simulink model "flightSim_Simulink"  (R2025b)
settings: Solver=VariableStepAuto  StartTime=0.0  StopTime=200  FixedStep=1/120  RelTol=1e-5
model workspace (MATLAB code in the model file):
  | initialize6DOFSkyHogg;
values from neighbouring files (symbols this model uses):
  aircraft = aircraft.update()    [flightSim_createAircraft.m]    (also in in_class_createAircraft.m)
  control = @(alpha, q) K_alpha*(alpha_desired - alpha) + K_q*(q_desired - q)    [sp_cntrl_ex.m]
  q = rate(2,itr)    [in_class_coding.m]    (also in in_class_sp_control.m = x(2,i); rigidBodyModel.m = rate(2); sp_cntrl_ex.m = xx(2,i))
  r = rate(3,itr)    [in_class_coding.m]    (also in rigidBodyModel.m = rate(3))
  state = fixedWingState(aircraft, Environment)    [flightSim_createAircraft.m]    (also in in_class_createAircraft.m)
undefined symbols (not defined in the file or in its folder): F, Light, MIL
libraries: aerolibasang x5, aerolibobsolete x1, aerolibadyn x1, aerolibatmos2 x1, aerolibwind2 x1, sharedtransform x1
settings Model: Creator=User  LastModifiedBy=tkhamvil
settings SolverCC: AlgebraicLoopSolver=TrustRegion  AutoInsertRateTranBlk=on  InsertRTBMode=Never (minimum delay)  MinimalZcImpactIntegration=on  MaxZcPerStep=1.0
settings DataIOCC: ExternalInput=inputs0  InitialState=states  SaveFormat=Array  SaveOutput=off
settings OptimizationCC: EnhancedBackFolding=on  StrengthReduction=on  InitFltsAndDblsToZero=on  DifferentSizesBufferReuse=on
settings DebuggingCC: WriteAfterWriteMsg=DisableAll  AlgebraicLoopMsg=none  FcnCallInpInsideContextMsg=warning  UniqueDataStoreMsg=error  RootOutportRequireBusObject=none  StateNameClashWarn=warning  StrictBusMsg=ErrorOnBusTreatedAsVector  SFUnexpectedBacktrackingDiag=warning  SFNoUnconditionalDefaultTransitionDiag=warning  SFExecutionAtInitializationDiag=none  ArithmeticOperatorsInVariantConditions=warning
settings ModelReferenceCC: EnableRefExpFcnMdlSchedulingChecks=on  PropagateSignalLabelsOutOfModel=off
settings SFSimCC: SimUseLocalCustomCode=off
settings RTWCC: RTWUseLocalCustomCode=off  GPUComputeCapability=3.5  DLArmComputeVersion=19.05
settings CodeAppCC: StateflowObjectComments=on

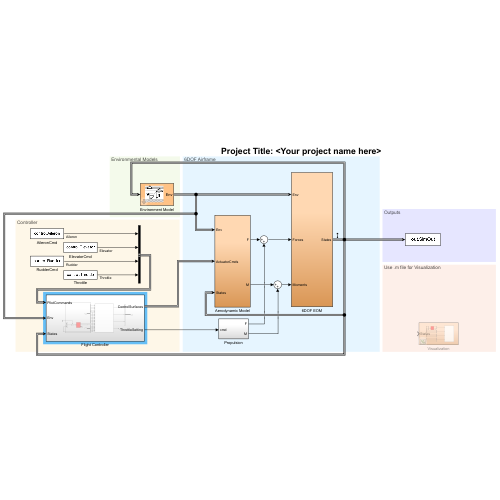
[thumbnail: Simulink's stored preview of the top-level diagram]
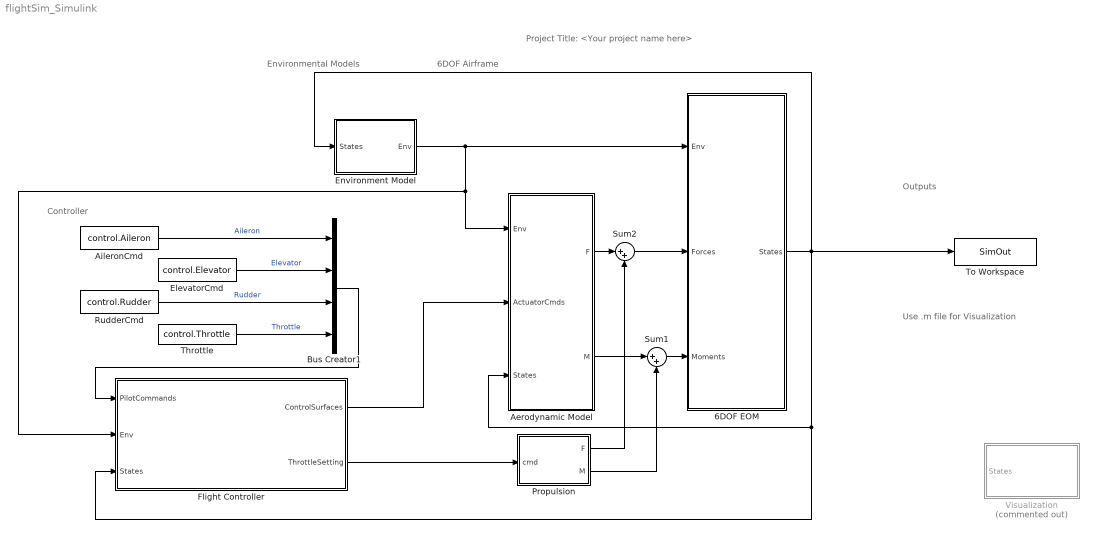
== system flightSim_Simulink ==
  note: Project Title: <Your project name here>
  note: 6DOF Airframe
  note: Environmental Models
  note: Controller
  note: Use .m file for Visualization
  note: Outputs
  6DOF EOM : Subsystem  VariantControl=eom3DOF
  Aerodynamic Model : Subsystem  VariantControl=aeroCONST
  AileronCmd : Constant  Value=control.Aileron
  Bus Creator1 : BusCreator  Inputs=4
  ElevatorCmd : Constant  Value=control.Elevator
  Environment Model : Subsystem  mask(Environment Model){spec=MIL-F-8785C, model=Continuous Dryden (+q -r), W20=5, Wdeg=0, TurbProb=10^-2 - Light, L_high=533.4, Wingspan=4, ts=0.1, Seed=[23341 23342 23343 23344], T_on=off, refAlt=state.GroundHeight}
      mask prompts: spec "aeroblks:aeroblkwind:blockWindTurbulenceModelParamSpecification"; model "aeroblks:aeroblkwind:blockWindTurbulenceModelParamModeltype"; W20 "Wind speed at 6 m defines the low-altitude intensity (m/s):"; Wdeg "Wind direction at 6 m (degrees clockwise from north):"; TurbProb "aeroblks:aeroblkwind:blockWindTurbulenceModelParamProbabilityofexceedanceofhighaltitudeintensity"; L_high "Scale length at medium/high altitudes (m):"; Wingspan "Wingspan (m):"; ts "Band limited noise sample time (sec):"; Seed "aeroblks:aeroblkwind:blockWindTurbulenceModelParamNoiseseedsugvgwgpg"; T_on "aeroblks:aeroblkwind:blockWindTurbulenceModelParamTurbulenceon"; refAlt "Reference height from Earth's surface to Flat Earth frame [m]:"
      mask help: This block contains an athmospheric model, a wind turbulence model, and a gravity model.
      mask Help: helpview(fullfile(docroot,'toolbox','aeroblks','aeroblks.map'), 'environment1');
      mask TypeOptions spec:
      | Dryden Wind Turbulence Model
      | (Continuous (+q +r))/spec
      mask TypeOptions model:
      | Dryden Wind Turbulence Model
      | (Continuous (+q +r))/model
      mask TypeOptions W20:
      | Dryden Wind Turbulence Model
      | (Continuous (+q +r))/W20
      mask TypeOptions Wdeg:
      | Dryden Wind Turbulence Model
      | (Continuous (+q +r))/Wdeg
      mask TypeOptions TurbProb:
      | Dryden Wind Turbulence Model
      | (Continuous (+q +r))/TurbProb
      mask TypeOptions L_high:
      | Dryden Wind Turbulence Model
      | (Continuous (+q +r))/L_high
      mask TypeOptions Wingspan:
      | Dryden Wind Turbulence Model
      | (Continuous (+q +r))/Wingspan
      mask TypeOptions ts:
      | Dryden Wind Turbulence Model
      | (Continuous (+q +r))/ts
      mask TypeOptions Seed:
      | Dryden Wind Turbulence Model
      | (Continuous (+q +r))/Seed
      mask TypeOptions T_on:
      | Dryden Wind Turbulence Model
      | (Continuous (+q +r))/T_on
      mask DialogControl Container4 Prompt: Atmospheric Model
      mask DialogControl Container17 Prompt: 1976 COESA-extended U.S. Standard Atmospheric Model
      mask DialogControl Control6 Prompt: There are no modifiable parameters for COESA.
      mask DialogControl Container6 Prompt: Wind Model
      mask DialogControl Container16 Prompt: Dryden Wind Turbulence Model
      mask DialogControl spec Prompt: Specification:
      mask DialogControl model Prompt: Model type:
      mask DialogControl TurbProb Prompt: Probability of exceedance of high-altitude intensity:
      mask DialogControl Seed Prompt: Noise seeds [ug vg wg pg]:
      mask DialogControl T_on Prompt: Turbulence on
      mask DialogControl Container8 Prompt: Gravity Model
      mask DialogControl Container18 Prompt: World Geodetic System (WGS 84) Gravity Taylor Series Model
      mask Display:
      | image('aeroenvironment.bmp',[.15,.15,.55,.75])
      | port_label('output',1,'Env')
  Flight Controller : Subsystem
  Propulsion : Subsystem
      settings: RTWSystemCode=Inline
  RudderCmd : Constant  Value=control.Rudder
  Sum1 : Sum  Inputs=|++  InputSameDT=on  SaturateOnIntegerOverflow=on  OutDataTypeStr=Inherit: Same as first input
  Sum2 : Sum  Inputs=|++  InputSameDT=on  SaturateOnIntegerOverflow=on  OutDataTypeStr=Inherit: Same as first input
  Throttle : Constant  Value=control.Throttle
  To Workspace : ToWorkspace  VariableName=SimOut  SaveFormat=Timeseries  SampleTime=-1
  Visualization : Subsystem  Commented=on
  wires:
  Sum2/1 -> 6DOF EOM/2(Forces)
  Propulsion/2(M) -> Sum1/2
  Propulsion/1(F) -> Sum2/2
  Sum1/1 -> 6DOF EOM/3(Moments)
  Aerodynamic Model/1(F) -> Sum2/1
  Aerodynamic Model/2(M) -> Sum1/1
  Environment Model/1(Env) -> Aerodynamic Model/1(Env), Flight Controller/2(Env), 6DOF EOM/1(Env)
  6DOF EOM/1(States) -> Flight Controller/3(States), Aerodynamic Model/3(States), To Workspace/1, Environment Model/1(States)
  Flight Controller/1(ControlSurfaces) -> Aerodynamic Model/2(ActuatorCmds)
  Flight Controller/2(ThrottleSetting) -> Propulsion/1(cmd)
  AileronCmd/1 -> Bus Creator1/1  "Aileron"
  ElevatorCmd/1 -> Bus Creator1/2  "Elevator"
  RudderCmd/1 -> Bus Creator1/3  "Rudder"
  Throttle/1 -> Bus Creator1/4  "Throttle"
  Bus Creator1/1 -> Flight Controller/1(PilotCommands)

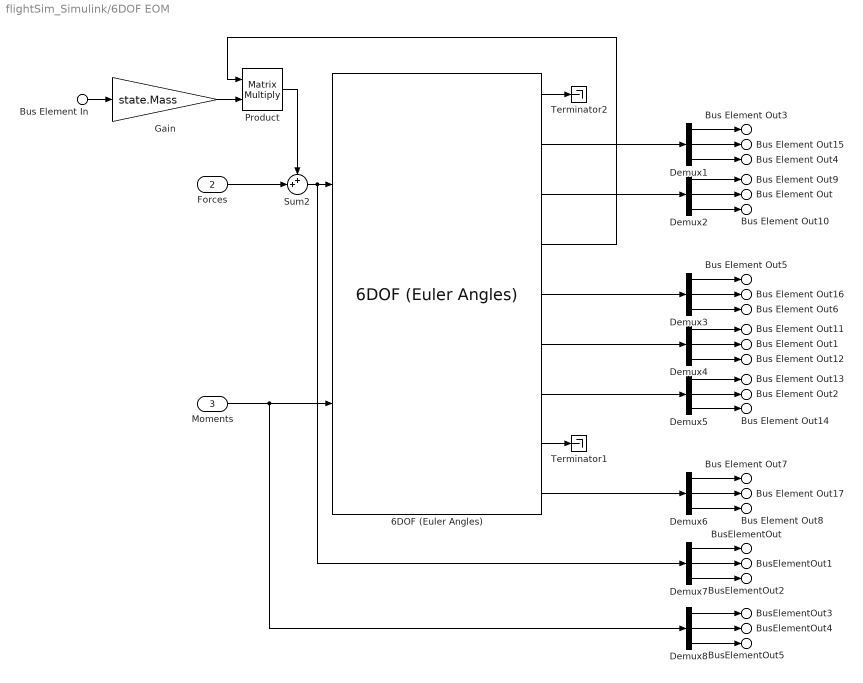
== system flightSim_Simulink/6DOF EOM ==
  Bus Element In : Inport  PortName=Env  Element=g
  Forces : Inport  Port=2
  Moments : Inport  Port=3
  6DOF (Euler Angles) : aerolibobsolete/6DOF (Euler Angles)  units=Metric (MKS)  mtype=Fixed  rep=Euler Angles  xme_0=[state.XN, state.XE, state.XD]  Vm_0=[state.U, state.V, state.W]  eul_0=[state.Phi, state.Theta, state.Psi]  pm_0=[state.P, state.Q, state.R]  mass_0=state.Mass  mass_e=0.5  mass_f=2.0  inertia=state.Inertia.Variables  inertia_e=eye(3)  inertia_f=2*eye(3)  k_quat=1.0  vre_flag=on  abi_flag=on  aMode=0  xme_statename={'Xe', 'Ye', 'Ze'}  Vm_statename={'U', 'V', 'W'}  eul_statename={'phi', 'theta', 'psi'}  quat_statename={'qr', 'qi', 'qj','qk'}  pm_statename={'p', 'q', 'r'}  mass_statename=''
  Demux{1..8} (8 alike) : Demux  Outputs=3
  Gain : Gain  Gain=state.Mass
  Product : Product  Multiplication=Matrix(*)
  Sum2 : Sum  Inputs=++|  InputSameDT=on  SaturateOnIntegerOverflow=on  OutDataTypeStr=Inherit: Same as first input
  Terminator1 : Terminator
  Terminator2 : Terminator
  Bus Element Out3 : Outport  VectorParamsAs1DForOutWhenUnconnected=off  PortName=States  Element=Xe
  Bus Element Out4 : Outport  VectorParamsAs1DForOutWhenUnconnected=off  PortName=States  Element=Ze
  Bus Element Out : Outport  VectorParamsAs1DForOutWhenUnconnected=off  PortName=States  Element=theta
  Bus Element Out5 : Outport  VectorParamsAs1DForOutWhenUnconnected=off  PortName=States  Element=u
  Bus Element Out6 : Outport  VectorParamsAs1DForOutWhenUnconnected=off  PortName=States  Element=w
  Bus Element Out1 : Outport  VectorParamsAs1DForOutWhenUnconnected=off  PortName=States  Element=q
  Bus Element Out2 : Outport  VectorParamsAs1DForOutWhenUnconnected=off  PortName=States  Element=q_dot
  Bus Element Out7 : Outport  VectorParamsAs1DForOutWhenUnconnected=off  PortName=States  Element=Axe
  Bus Element Out8 : Outport  VectorParamsAs1DForOutWhenUnconnected=off  PortName=States  Element=Aze
  Bus Element Out15 : Outport  VectorParamsAs1DForOutWhenUnconnected=off  PortName=States  Element=Ye
  Bus Element Out9 : Outport  VectorParamsAs1DForOutWhenUnconnected=off  PortName=States  Element=phi
  Bus Element Out10 : Outport  VectorParamsAs1DForOutWhenUnconnected=off  PortName=States  Element=psi
  Bus Element Out16 : Outport  VectorParamsAs1DForOutWhenUnconnected=off  PortName=States  Element=v
  Bus Element Out11 : Outport  VectorParamsAs1DForOutWhenUnconnected=off  PortName=States  Element=p
  Bus Element Out12 : Outport  VectorParamsAs1DForOutWhenUnconnected=off  PortName=States  Element=r
  Bus Element Out13 : Outport  VectorParamsAs1DForOutWhenUnconnected=off  PortName=States  Element=p_dot
  Bus Element Out14 : Outport  VectorParamsAs1DForOutWhenUnconnected=off  PortName=States  Element=r_dot
  Bus Element Out17 : Outport  VectorParamsAs1DForOutWhenUnconnected=off  PortName=States  Element=Aye
  BusElementOut : Outport  PortName=States  Element=X
  BusElementOut1 : Outport  PortName=States  Element=Y
  BusElementOut2 : Outport  PortName=States  Element=Z
  BusElementOut3 : Outport  PortName=States  Element=L
  BusElementOut4 : Outport  PortName=States  Element=M
  BusElementOut5 : Outport  PortName=States  Element=N
  wires:
  6DOF (Euler Angles)/2 -> Demux1/1
  6DOF (Euler Angles)/4 -> Product/1
  6DOF (Euler Angles)/1 -> Terminator2/1
  Bus Element In/1 -> Gain/1
  Demux6/2 -> Bus Element Out17/1
  Demux6/3 -> Bus Element Out8/1
  Demux6/1 -> Bus Element Out7/1
  6DOF (Euler Angles)/9 -> Demux6/1
  6DOF (Euler Angles)/7 -> Demux5/1
  Demux5/3 -> Bus Element Out14/1
  Demux5/2 -> Bus Element Out2/1
  Demux5/1 -> Bus Element Out13/1
  6DOF (Euler Angles)/6 -> Demux4/1
  Demux4/3 -> Bus Element Out12/1
  Demux4/2 -> Bus Element Out1/1
  Demux4/1 -> Bus Element Out11/1
  Demux3/3 -> Bus Element Out6/1
  Demux3/2 -> Bus Element Out16/1
  Demux3/1 -> Bus Element Out5/1
  6DOF (Euler Angles)/5 -> Demux3/1
  Demux2/3 -> Bus Element Out10/1
  Demux2/2 -> Bus Element Out/1
  Demux2/1 -> Bus Element Out9/1
  Demux1/1 -> Bus Element Out3/1
  Demux1/3 -> Bus Element Out4/1
  Demux1/2 -> Bus Element Out15/1
  Gain/1 -> Product/2
  6DOF (Euler Angles)/3 -> Demux2/1
  Forces/1 -> Sum2/2
  Product/1 -> Sum2/1
  6DOF (Euler Angles)/8 -> Terminator1/1
  Sum2/1 -> Demux7/1, 6DOF (Euler Angles)/1
  Moments/1 -> Demux8/1, 6DOF (Euler Angles)/2
  Demux7/1 -> BusElementOut/1
  Demux7/2 -> BusElementOut1/1
  Demux7/3 -> BusElementOut2/1
  Demux8/1 -> BusElementOut3/1
  Demux8/2 -> BusElementOut4/1
  Demux8/3 -> BusElementOut5/1

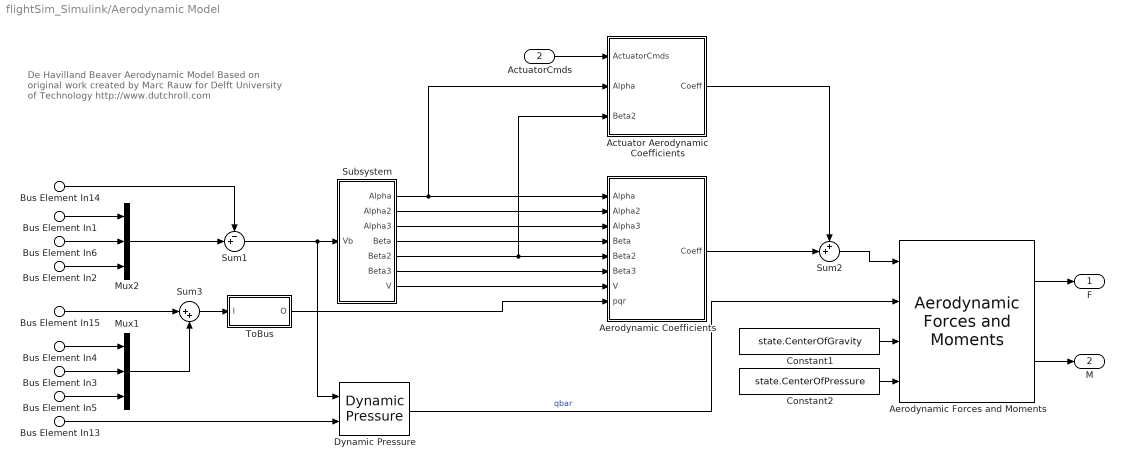
== system flightSim_Simulink/Aerodynamic Model ==
  note: De Havilland Beaver Aerodynamic Model
      | Based on original work created by
      | Marc Rauw for Delft University of Technology
      | http://www.dutchroll.com
  Bus Element In13 : Inport  PortName=Env  Element=AirDensity
  Bus Element In14 : Inport  PortName=Env  Element=WindVelocity
  Bus Element In15 : Inport  PortName=Env  Element=WindAngularRates
  ActuatorCmds : Inport  Port=2
  Bus Element In1 : Inport  Port=3  PortName=States  Element=u
  Bus Element In2 : Inport  Port=3  PortName=States  Element=w
  Bus Element In3 : Inport  Port=3  PortName=States  Element=q
  Bus Element In6 : Inport  Port=3  PortName=States  Element=v
  Bus Element In4 : Inport  Port=3  PortName=States  Element=p
  Bus Element In5 : Inport  Port=3  PortName=States  Element=r
  Actuator Aerodynamic Coefficients : Subsystem
  Aerodynamic Coefficients : Subsystem
  Aerodynamic Forces and Moments : aerolibadyn/Aerodynamic Forces and Moments   inputAxes=Body  outputForceAxes=Body  outputMomentAxes=Body  S=aircraft.ReferenceArea  b=aircraft.ReferenceSpan  cbar=aircraft.ReferenceLength
  Constant1 : Constant  Value=state.CenterOfGravity
  Constant2 : Constant  Value=state.CenterOfPressure
  Dynamic Pressure : aerolibasang/Dynamic Pressure
  Mux1 : Mux  Inputs=3
  Mux2 : Mux  Inputs=3
  Subsystem : Subsystem
  Sum1 : Sum  Inputs=-+|  InputSameDT=on  SaturateOnIntegerOverflow=on  OutDataTypeStr=Inherit: Same as first input
  Sum2 : Sum  Inputs=++|
  Sum3 : Sum  Inputs=|++  InputSameDT=on  SaturateOnIntegerOverflow=on  OutDataTypeStr=Inherit: Same as first input
  ToBus : Subsystem
  F : Outport  Unit=N  VectorParamsAs1DForOutWhenUnconnected=off
  M : Outport  Port=2  Unit=N*m  VectorParamsAs1DForOutWhenUnconnected=off
  wires:
  ActuatorCmds/1 -> Actuator Aerodynamic Coefficients/1(ActuatorCmds)
  Bus Element In14/1 -> Sum1/1
  Mux2/1 -> Sum1/2
  Mux1/1 -> Sum3/2
  Bus Element In15/1 -> Sum3/1
  Bus Element In5/1 -> Mux1/3
  Bus Element In3/1 -> Mux1/2
  Bus Element In4/1 -> Mux1/1
  Actuator Aerodynamic Coefficients/1(Coeff) -> Sum2/1
  Aerodynamic Coefficients/1(Coeff) -> Sum2/2
  ToBus/1(O) -> Aerodynamic Coefficients/8(pqr)
  Sum1/1 -> Dynamic Pressure/1, Subsystem/1(Vb)
  Dynamic Pressure/1 -> Aerodynamic Forces and Moments/2  "qbar"
  Sum3/1 -> ToBus/1(I)
  Bus Element In13/1 -> Dynamic Pressure/2
  Subsystem/7(V) -> Aerodynamic Coefficients/7(V)
  Subsystem/4(Beta) -> Aerodynamic Coefficients/4(Beta)
  Aerodynamic Forces and Moments/2 -> M/1
  Aerodynamic Forces and Moments/1 -> F/1
  Constant2/1 -> Aerodynamic Forces and Moments/4
  Constant1/1 -> Aerodynamic Forces and Moments/3
  Sum2/1 -> Aerodynamic Forces and Moments/1
  Bus Element In1/1 -> Mux2/1
  Bus Element In6/1 -> Mux2/2
  Bus Element In2/1 -> Mux2/3
  Subsystem/1(Alpha) -> Aerodynamic Coefficients/1(Alpha), Actuator Aerodynamic Coefficients/2(Alpha)
  Subsystem/5(Beta2) -> Aerodynamic Coefficients/5(Beta2), Actuator Aerodynamic Coefficients/3(Beta2)
  Subsystem/2(Alpha2) -> Aerodynamic Coefficients/2(Alpha2)
  Subsystem/3(Alpha3) -> Aerodynamic Coefficients/3(Alpha3)
  Subsystem/6(Beta3) -> Aerodynamic Coefficients/6(Beta3)

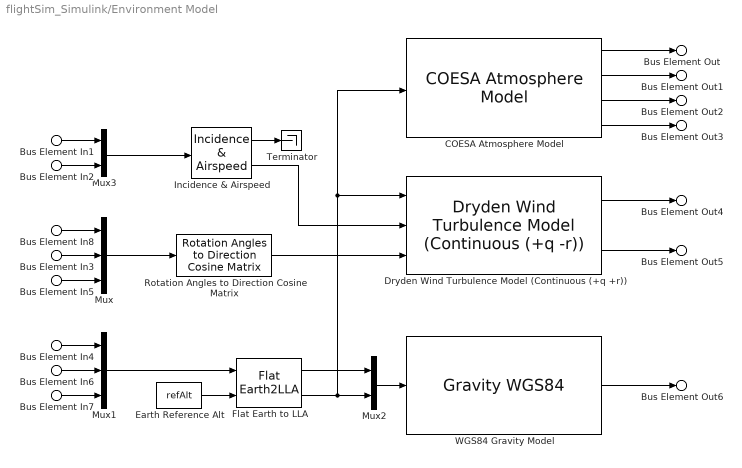
== system flightSim_Simulink/Environment Model ==
  Bus Element In1 : Inport  PortName=States  Element=u
  Bus Element In2 : Inport  PortName=States  Element=w
  Bus Element In3 : Inport  PortName=States  Element=theta
  Bus Element In4 : Inport  PortName=States  Element=Xe
  Bus Element In7 : Inport  PortName=States  Element=Ze
  Bus Element In8 : Inport  PortName=States  Element=phi
  Bus Element In5 : Inport  PortName=States  Element=psi
  Bus Element In6 : Inport  PortName=States  Element=Ye
  COESA Atmosphere Model : aerolibatmos2/COESA Atmosphere Model  units=Metric (MKS)  spec=1976 COESA-extended U.S. Standard Atmosphere  model=Profile  profile_var=High temperature  profile_percent=1%  profile_alt=5 km (16404 ft)  envelope_var=High temperature  envelope_percent=1%  action=Warning
  Dryden Wind Turbulence Model (Continuous (+q +r)) : aerolibwind2/Dryden Wind Turbulence Model  (Continuous (+q -r))  units=Metric (MKS)  spec=MIL-F-8785C  model=Continuous Dryden (+q -r)  W20=W20  Wdeg=Wdeg  TurbProb=10^-2 - Light  L_high=L_high  Wingspan=Wingspan  ts=ts  Seed=Seed  T_on=off
  Earth Reference Alt : Constant  Value=refAlt
  Flat Earth to LLA : FlatEarth2LLA  R=6378137  LL0=[0 0]
  Incidence & Airspeed : aerolibasang/Incidence  & Airspeed
  Mux : Mux  Inputs=3
  Mux1 : Mux  Inputs=3
  Mux2 : Mux  Inputs=2
  Mux3 : Mux  Inputs=2
  Rotation Angles to Direction Cosine Matrix : sharedtransform/Rotation Angles to Direction Cosine Matrix  rotationOrder=ZYX  aMode=aMode
  Terminator : Terminator
  "WGS84 Gravity Model  " : GravityWGS84
  Bus Element Out : Outport  VectorParamsAs1DForOutWhenUnconnected=off  PortName=Env  Element=To
  Bus Element Out1 : Outport  VectorParamsAs1DForOutWhenUnconnected=off  PortName=Env  Element=a
  Bus Element Out2 : Outport  VectorParamsAs1DForOutWhenUnconnected=off  PortName=Env  Element=Po
  Bus Element Out3 : Outport  VectorParamsAs1DForOutWhenUnconnected=off  PortName=Env  Element=AirDensity
  Bus Element Out4 : Outport  VectorParamsAs1DForOutWhenUnconnected=off  PortName=Env  Element=WindVelocity
  Bus Element Out5 : Outport  VectorParamsAs1DForOutWhenUnconnected=off  PortName=Env  Element=WindAngularRates
  Bus Element Out6 : Outport  VectorParamsAs1DForOutWhenUnconnected=off  PortName=Env  Element=g
  wires:
  Dryden Wind Turbulence Model (Continuous (+q +r))/1 -> Bus Element Out4/1
  Dryden Wind Turbulence Model (Continuous (+q +r))/2 -> Bus Element Out5/1
  Mux2/1 -> "WGS84 Gravity Model  "/1
  Bus Element In4/1 -> Mux1/1
  Bus Element In7/1 -> Mux1/3
  Bus Element In6/1 -> Mux1/2
  Bus Element In5/1 -> Mux/3
  Bus Element In8/1 -> Mux/1
  Bus Element In2/1 -> Mux3/2
  Bus Element In1/1 -> Mux3/1
  "WGS84 Gravity Model  "/1 -> Bus Element Out6/1
  COESA Atmosphere Model/2 -> Bus Element Out1/1
  COESA Atmosphere Model/1 -> Bus Element Out/1
  COESA Atmosphere Model/4 -> Bus Element Out3/1
  COESA Atmosphere Model/3 -> Bus Element Out2/1
  Flat Earth to LLA/1 -> Mux2/1
  Earth Reference Alt/1 -> Flat Earth to LLA/2
  Incidence & Airspeed/2 -> Dryden Wind Turbulence Model (Continuous (+q +r))/2
  Flat Earth to LLA/2 -> Mux2/2, COESA Atmosphere Model/1, Dryden Wind Turbulence Model (Continuous (+q +r))/1
  Mux3/1 -> Incidence & Airspeed/1
  Incidence & Airspeed/1 -> Terminator/1
  Mux/1 -> Rotation Angles to Direction Cosine Matrix/1
  Bus Element In3/1 -> Mux/2
  Rotation Angles to Direction Cosine Matrix/1 -> Dryden Wind Turbulence Model (Continuous (+q +r))/3
  Mux1/1 -> Flat Earth to LLA/1

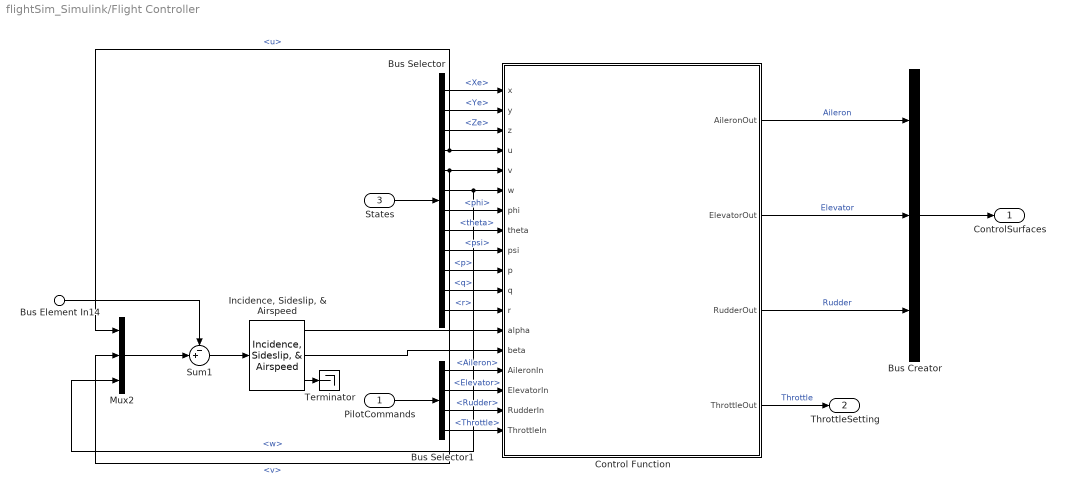
== system flightSim_Simulink/Flight Controller ==
  PilotCommands : Inport
  Bus Element In14 : Inport  Port=2  PortName=Env  Element=WindVelocity
  States : Inport  Port=3
  Bus Creator : BusCreator  Inputs=3
  Bus Selector : BusSelector  OutputSignals=Xe,Ye,Ze,u,v,w,phi,theta,psi,p,q,r
  Bus Selector1 : BusSelector  OutputSignals=Aileron,Elevator,Rudder,Throttle
  Control Function : MATLAB Function  TreatAsAtomicUnit=on
  "Incidence, Sideslip, & Airspeed" : aerolibasang/Incidence, Sideslip, & Airspeed
  Mux2 : Mux  Inputs=3
  Sum1 : Sum  Inputs=-+|  InputSameDT=on  SaturateOnIntegerOverflow=on  OutDataTypeStr=Inherit: Same as first input
  Terminator : Terminator
  ControlSurfaces : Outport
  ThrottleSetting : Outport  Port=2
  wires:
  Control Function/1(AileronOut) -> Bus Creator/1  "Aileron"
  Bus Creator/1 -> ControlSurfaces/1
  States/1 -> Bus Selector/1
  Bus Selector/1 -> Control Function/1(x)  "<Xe>"
  Bus Selector/2 -> Control Function/2(y)  "<Ye>"
  Bus Selector/3 -> Control Function/3(z)  "<Ze>"
  Bus Selector/4 -> Control Function/4(u), Mux2/1  "<u>"
  Bus Selector/5 -> Control Function/5(v), Mux2/2  "<v>"
  Bus Selector/6 -> Control Function/6(w), Mux2/3  "<w>"
  Bus Selector/7 -> Control Function/7(phi)  "<phi>"
  Bus Selector/8 -> Control Function/8(theta)  "<theta>"
  Bus Selector/9 -> Control Function/9(psi)  "<psi>"
  Bus Selector/10 -> Control Function/10(p)  "<p>"
  Bus Selector/11 -> Control Function/11(q)  "<q>"
  Bus Selector/12 -> Control Function/12(r)  "<r>"
  PilotCommands/1 -> Bus Selector1/1
  Bus Selector1/1 -> Control Function/15(AileronIn)  "<Aileron>"
  Bus Selector1/4 -> Control Function/18(ThrottleIn)  "<Throttle>"
  Bus Selector1/3 -> Control Function/17(RudderIn)  "<Rudder>"
  Bus Selector1/2 -> Control Function/16(ElevatorIn)  "<Elevator>"
  Control Function/2(ElevatorOut) -> Bus Creator/2  "Elevator"
  Control Function/3(RudderOut) -> Bus Creator/3  "Rudder"
  Control Function/4(ThrottleOut) -> ThrottleSetting/1  "Throttle"
  Bus Element In14/1 -> Sum1/1
  Mux2/1 -> Sum1/2
  Sum1/1 -> "Incidence, Sideslip, & Airspeed"/1
  "Incidence, Sideslip, & Airspeed"/3 -> Terminator/1
  "Incidence, Sideslip, & Airspeed"/2 -> Control Function/14(beta)
  "Incidence, Sideslip, & Airspeed"/1 -> Control Function/13(alpha)

== system flightSim_Simulink/Propulsion ==
  cmd : Inport
  Mux : Mux  Inputs=[1 2]
  ThrustX : Lookup_n-D  NumberOfTableDimensions=1  DataSpecification=Lookup table object  LookupTableObject=thrustX  BreakpointsForDimension1="getCoefficient(aircraft,\"CX\",\"Propeller\",Component=\"Propeller\").Breakpoints(1).Value"  IndexSearchMethod=Linear search  BeginIndexSearchUsingPreviousIndexResult=on  Table="getCoefficient(aircraft,\"CX\",\"Propeller\",Component=\"Propeller\").Table.Value"  ExtrapMethod=Clip
  ThrustYZ : Constant  Value=[0 0]'  SampleTime=-1
  Thrust_M1 : Constant  Value=[0 0 0]'  SampleTime=-1
  F : Outport  Unit=N  VectorParamsAs1DForOutWhenUnconnected=off
  M : Outport  Port=2  Unit=N*m  VectorParamsAs1DForOutWhenUnconnected=off
  wires:
  Thrust_M1/1 -> M/1
  ThrustX/1 -> Mux/1
  ThrustYZ/1 -> Mux/2
  Mux/1 -> F/1
  cmd/1 -> ThrustX/1

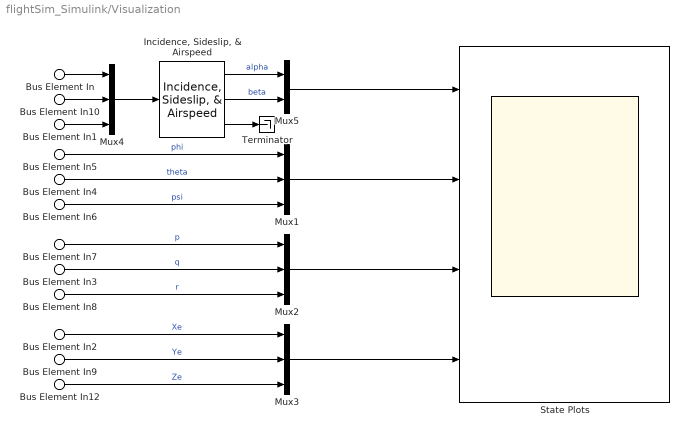
== system flightSim_Simulink/Visualization ==
  Bus Element In : Inport  PortName=States  Element=u
  Bus Element In1 : Inport  PortName=States  Element=w
  Bus Element In3 : Inport  PortName=States  Element=q
  Bus Element In4 : Inport  PortName=States  Element=theta
  Bus Element In12 : Inport  PortName=States  Element=Ze
  Bus Element In2 : Inport  PortName=States  Element=Xe
  Bus Element In10 : Inport  PortName=States  Element=v
  Bus Element In5 : Inport  PortName=States  Element=phi
  Bus Element In6 : Inport  PortName=States  Element=psi
  Bus Element In7 : Inport  PortName=States  Element=p
  Bus Element In8 : Inport  PortName=States  Element=r
  Bus Element In9 : Inport  PortName=States  Element=Ye
  "Incidence, Sideslip, & Airspeed" : aerolibasang/Incidence, Sideslip, & Airspeed
  Mux{1..4} (4 alike) : Mux  Inputs=3
  Mux5 : Mux  Inputs=2
  State Plots : Scope  NumInputPorts=4
      settings: Title=Incidence and Sideslip Angle vs Time  ActiveDisplayYMinimum=0.02467  ActiveDisplayYMaximum=0.15024  YLabel=\alpha \beta [rad]
  Terminator : Terminator
  wires:
  Mux3/1 -> State Plots/4
  Bus Element In2/1 -> Mux3/1  "Xe"
  Bus Element In9/1 -> Mux3/2  "Ye"
  Bus Element In12/1 -> Mux3/3  "Ze"
  Mux2/1 -> State Plots/3
  Mux1/1 -> State Plots/2
  Mux5/1 -> State Plots/1
  "Incidence, Sideslip, & Airspeed"/2 -> Mux5/2  "beta"
  "Incidence, Sideslip, & Airspeed"/1 -> Mux5/1  "alpha"
  Mux4/1 -> "Incidence, Sideslip, & Airspeed"/1
  Bus Element In10/1 -> Mux4/2
  Bus Element In8/1 -> Mux2/3  "r"
  Bus Element In7/1 -> Mux2/1  "p"
  Bus Element In6/1 -> Mux1/3  "psi"
  Bus Element In5/1 -> Mux1/1  "phi"
  Bus Element In4/1 -> Mux1/2  "theta"
  Bus Element In3/1 -> Mux2/2  "q"
  Bus Element In1/1 -> Mux4/3
  Bus Element In/1 -> Mux4/1
  "Incidence, Sideslip, & Airspeed"/3 -> Terminator/1

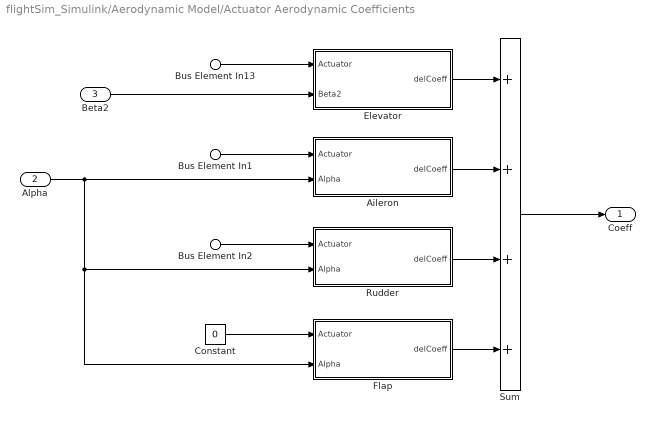
== system flightSim_Simulink/Aerodynamic Model/Actuator Aerodynamic Coefficients ==
  Bus Element In13 : Inport  PortName=ActuatorCmds  Element=Elevator
  Bus Element In1 : Inport  PortName=ActuatorCmds  Element=Aileron
  Bus Element In2 : Inport  PortName=ActuatorCmds  Element=Rudder
  Alpha : Inport  Port=2
  Beta2 : Inport  Port=3
  Aileron : Subsystem
  Constant : Constant  Value=0
  Elevator : Subsystem
  Flap : Subsystem
  Rudder : Subsystem
  Sum : Sum  Inputs=4  InputSameDT=on  SaturateOnIntegerOverflow=on  OutDataTypeStr=Inherit: Same as first input
  Coeff : Outport  InitialOutput=0  VectorParamsAs1DForOutWhenUnconnected=off
  wires:
  Constant/1 -> Flap/1(Actuator)
  Bus Element In2/1 -> Rudder/1(Actuator)
  Bus Element In1/1 -> Aileron/1(Actuator)
  Bus Element In13/1 -> Elevator/1(Actuator)
  Beta2/1 -> Elevator/2(Beta2)
  Flap/1(delCoeff) -> Sum/4
  Alpha/1 -> Flap/2(Alpha), Rudder/2(Alpha), Aileron/2(Alpha)
  Rudder/1(delCoeff) -> Sum/3
  Aileron/1(delCoeff) -> Sum/2
  Elevator/1(delCoeff) -> Sum/1
  Sum/1 -> Coeff/1

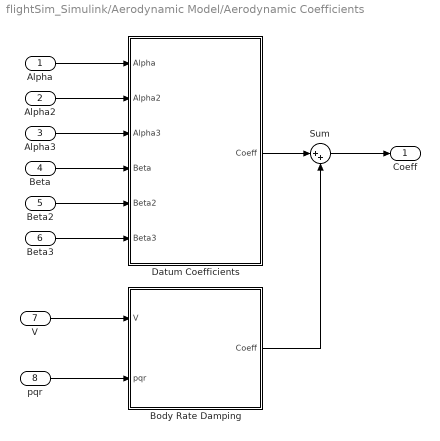
== system flightSim_Simulink/Aerodynamic Model/Aerodynamic Coefficients ==
  Alpha : Inport
  Alpha2 : Inport  Port=2
  Alpha3 : Inport  Port=3
  Beta : Inport  Port=4
  Beta2 : Inport  Port=5
  Beta3 : Inport  Port=6
  V : Inport  Port=7
  pqr : Inport  Port=8  Unit=m/s
  Body Rate Damping : Subsystem
  Datum Coefficients : Subsystem
  Sum : Sum  Inputs=|++
  Coeff : Outport  VectorParamsAs1DForOutWhenUnconnected=off
  wires:
  pqr/1 -> Body Rate Damping/2(pqr)
  Sum/1 -> Coeff/1
  V/1 -> Body Rate Damping/1(V)
  Body Rate Damping/1(Coeff) -> Sum/2
  Datum Coefficients/1(Coeff) -> Sum/1
  Beta/1 -> Datum Coefficients/4(Beta)
  Alpha/1 -> Datum Coefficients/1(Alpha)
  Alpha2/1 -> Datum Coefficients/2(Alpha2)
  Alpha3/1 -> Datum Coefficients/3(Alpha3)
  Beta2/1 -> Datum Coefficients/5(Beta2)
  Beta3/1 -> Datum Coefficients/6(Beta3)

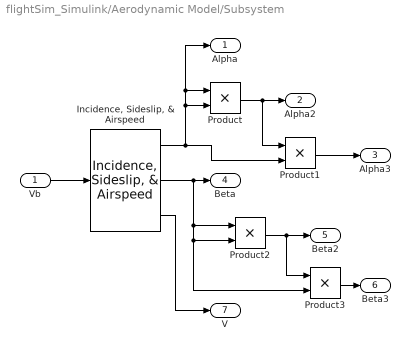
== system flightSim_Simulink/Aerodynamic Model/Subsystem ==
  Vb : Inport
  "Incidence, Sideslip, & Airspeed" : aerolibasang/Incidence, Sideslip, & Airspeed
  Product{,1..3} (4 alike) : Product
  Alpha : Outport
  Alpha2 : Outport  Port=2
  Alpha3 : Outport  Port=3
  Beta : Outport  Port=4
  Beta2 : Outport  Port=5
  Beta3 : Outport  Port=6
  V : Outport  Port=7
  wires:
  Product/1 -> Product1/1, Alpha2/1
  "Incidence, Sideslip, & Airspeed"/1 -> Product/1, Alpha/1, Product/2, Product1/2
  "Incidence, Sideslip, & Airspeed"/3 -> V/1
  Vb/1 -> "Incidence, Sideslip, & Airspeed"/1
  Product1/1 -> Alpha3/1
  Product2/1 -> Product3/1, Beta2/1
  Product3/1 -> Beta3/1
  "Incidence, Sideslip, & Airspeed"/2 -> Product3/2, Product2/2, Product2/1, Beta/1

== system flightSim_Simulink/Aerodynamic Model/ToBus ==
  I : Inport
  Bus Creator3 : BusCreator  Inputs=3
  Demux : Demux  Outputs=3
  O : Outport  VectorParamsAs1DForOutWhenUnconnected=off
  wires:
  I/1 -> Demux/1
  Demux/2 -> Bus Creator3/2  "q_wind"
  Bus Creator3/1 -> O/1
  Demux/3 -> Bus Creator3/3  "r_wind"
  Demux/1 -> Bus Creator3/1  "p_wind"

== system flightSim_Simulink/Aerodynamic Model/Actuator Aerodynamic Coefficients/Aileron ==
  Actuator : Inport
  Alpha : Inport  Port=2
  Constant : Constant  Value=aircraft.Surfaces(1).Surfaces(1).Coefficients.Table.Variables
  Matrix Multiply : Product  Multiplication=Matrix(*)
  Product : Product
  Vector Concatenate : Concatenate
  delCoeff : Outport  VectorParamsAs1DForOutWhenUnconnected=off
  wires:
  Actuator/1 -> Product/1, Vector Concatenate/1
  Alpha/1 -> Product/2
  Vector Concatenate/1 -> Matrix Multiply/2
  Matrix Multiply/1 -> delCoeff/1
  Product/1 -> Vector Concatenate/2
  Constant/1 -> Matrix Multiply/1

== system flightSim_Simulink/Aerodynamic Model/Actuator Aerodynamic Coefficients/Elevator ==
  Actuator : Inport
  Beta2 : Inport  Port=2
  Constant : Constant  Value=aircraft.Surfaces(2).Surfaces(1).Coefficients.Table.Variables
  Matrix Multiply : Product  Multiplication=Matrix(*)
  Product : Product
  Vector Concatenate : Concatenate
  delCoeff : Outport  VectorParamsAs1DForOutWhenUnconnected=off
  wires:
  Matrix Multiply/1 -> delCoeff/1
  Constant/1 -> Matrix Multiply/1
  Vector Concatenate/1 -> Matrix Multiply/2
  Actuator/1 -> Product/1, Vector Concatenate/1
  Beta2/1 -> Product/2
  Product/1 -> Vector Concatenate/2

== system flightSim_Simulink/Aerodynamic Model/Actuator Aerodynamic Coefficients/Flap ==
  Actuator : Inport
  Alpha : Inport  Port=2
  Constant : Constant  Value=aircraft.Surfaces(1).Surfaces(2).Coefficients.Table.Variables
  Matrix Multiply : Product  Multiplication=Matrix(*)
  Product : Product
  Vector Concatenate : Concatenate
  delCoeff : Outport  VectorParamsAs1DForOutWhenUnconnected=off
  wires:
  Actuator/1 -> Product/1, Vector Concatenate/1
  Alpha/1 -> Product/2
  Vector Concatenate/1 -> Matrix Multiply/2
  Matrix Multiply/1 -> delCoeff/1
  Product/1 -> Vector Concatenate/2
  Constant/1 -> Matrix Multiply/1

== system flightSim_Simulink/Aerodynamic Model/Actuator Aerodynamic Coefficients/Rudder ==
  Actuator : Inport
  Alpha : Inport  Port=2
  Constant : Constant  Value=aircraft.Surfaces(3).Surfaces(1).Coefficients.Table.Variables
  Matrix Multiply : Product  Multiplication=Matrix(*)
  Product : Product
  Vector Concatenate : Concatenate
  delCoeff : Outport  VectorParamsAs1DForOutWhenUnconnected=off
  wires:
  Actuator/1 -> Product/1, Vector Concatenate/1
  Alpha/1 -> Product/2
  Vector Concatenate/1 -> Matrix Multiply/2
  Matrix Multiply/1 -> delCoeff/1
  Product/1 -> Vector Concatenate/2
  Constant/1 -> Matrix Multiply/1

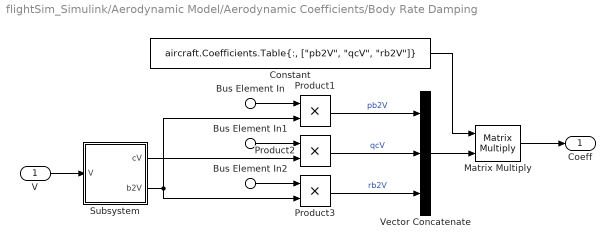
== system flightSim_Simulink/Aerodynamic Model/Aerodynamic Coefficients/Body Rate Damping ==
  V : Inport  Unit=m/s
  Bus Element In : Inport  Port=2  PortName=pqr  Element=p_wind
  Bus Element In1 : Inport  Port=2  PortName=pqr  Element=q_wind
  Bus Element In2 : Inport  Port=2  PortName=pqr  Element=r_wind
  Constant : Constant  Value="aircraft.Coefficients.Table{:, [\"pb2V\", \"qcV\", \"rb2V\"]}"
  Matrix Multiply : Product  Multiplication=Matrix(*)
  Product1 : Product
  Product2 : Product
  Product3 : Product
  Subsystem : Subsystem
  Vector Concatenate : Concatenate  NumInputs=3
  Coeff : Outport  InitialOutput=0  VectorParamsAs1DForOutWhenUnconnected=off
  wires:
  Matrix Multiply/1 -> Coeff/1
  Vector Concatenate/1 -> Matrix Multiply/2
  Product1/1 -> Vector Concatenate/1  "pb2V"
  Bus Element In/1 -> Product1/1
  Product2/1 -> Vector Concatenate/2  "qcV"
  Subsystem/2(b2V) -> Product3/2, Product1/2
  Product3/1 -> Vector Concatenate/3  "rb2V"
  Constant/1 -> Matrix Multiply/1
  Bus Element In1/1 -> Product2/1
  Subsystem/1(cV) -> Product2/2
  Bus Element In2/1 -> Product3/1
  V/1 -> Subsystem/1(V)

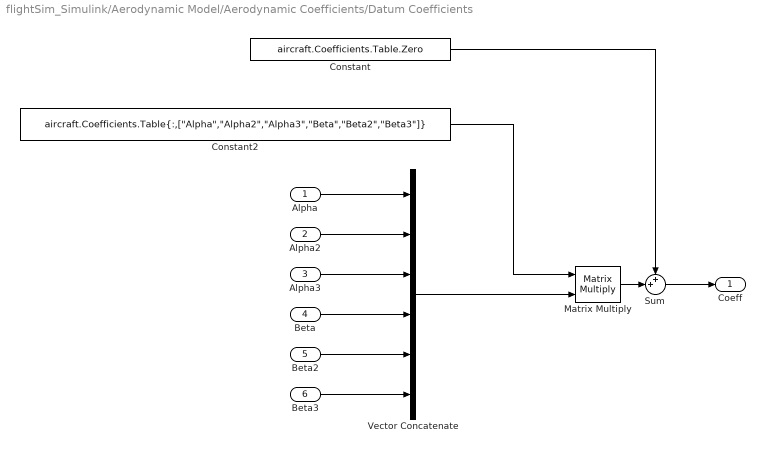
== system flightSim_Simulink/Aerodynamic Model/Aerodynamic Coefficients/Datum Coefficients ==
  Alpha : Inport
  Alpha2 : Inport  Port=2
  Alpha3 : Inport  Port=3
  Beta : Inport  Port=4
  Beta2 : Inport  Port=5
  Beta3 : Inport  Port=6
  Constant : Constant  Value=aircraft.Coefficients.Table.Zero
  Constant2 : Constant  Value="aircraft.Coefficients.Table{:,[\"Alpha\",\"Alpha2\",\"Alpha3\",\"Beta\",\"Beta2\",\"Beta3\"]}"
  Matrix Multiply : Product  Multiplication=Matrix(*)
  Sum : Sum  Inputs=++|
  Vector Concatenate : Concatenate  NumInputs=6
  Coeff : Outport  InitialOutput=0  VectorParamsAs1DForOutWhenUnconnected=off
  wires:
  Sum/1 -> Coeff/1
  Constant/1 -> Sum/1
  Matrix Multiply/1 -> Sum/2
  Alpha/1 -> Vector Concatenate/1
  Vector Concatenate/1 -> Matrix Multiply/2
  Constant2/1 -> Matrix Multiply/1
  Beta/1 -> Vector Concatenate/4
  Alpha3/1 -> Vector Concatenate/3
  Alpha2/1 -> Vector Concatenate/2
  Beta2/1 -> Vector Concatenate/5
  Beta3/1 -> Vector Concatenate/6

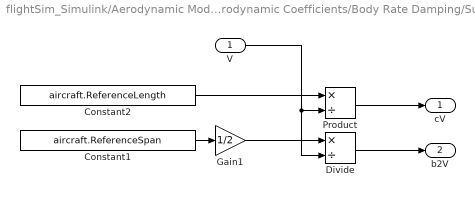
== system flightSim_Simulink/Aerodynamic Model/Aerodynamic Coefficients/Body Rate Damping/Subsystem ==
  V : Inport
  Constant1 : Constant  Value=aircraft.ReferenceSpan
  Constant2 : Constant  Value=aircraft.ReferenceLength
  Divide : Product  Inputs=*/
  Gain1 : Gain  Gain=1/2
  Product : Product  Inputs=*/
  cV : Outport
  b2V : Outport  Port=2
  wires:
  Product/1 -> cV/1
  Constant1/1 -> Gain1/1
  V/1 -> Divide/2, Product/2
  Divide/1 -> b2V/1
  Constant2/1 -> Product/1
  Gain1/1 -> Divide/1

== matlab function flightSim_Simulink/Flight Controller/Control Function ==
  data: AileronOut output; ElevatorOut output; x input double; y input; z input; u input; v input; w input; phi input; theta input; psi input; p input; q input; r input; alpha input; beta input; RudderOut output; ThrottleOut output; AileronIn input; ElevatorIn input; RudderIn input; ThrottleIn input
function [AileronOut, ElevatorOut, RudderOut, ThrottleOut] = flightController(x,y,z,u,v,w,phi,theta,psi,p,q,r,alpha,beta,AileronIn,ElevatorIn,RudderIn,ThrottleIn)
%% Pick one between manual and autopilot
goForAuto = 1;

if (~goForAuto) % Manual
    %% Manual Pilot Control
    AileronOut  = AileronIn;
    ElevatorOut = ElevatorIn;
    RudderOut   = RudderIn;
    ThrottleOut = ThrottleIn;
else % Autopilot
    %% Correct for Actuator Direction
    ua_in = -AileronIn;
    ue_in = -ElevatorIn;
    ur_in = -RudderIn;
    ut_in =  ThrottleIn;
    
    %% Examples Controllers (pick/add one)
    % rate SAS from trim condition
    % ua = -p + ua_in;
    % ue = -5*q + ue_in;
    % ur = -r + ur_in;
    % ut = ut_in;
    
    %- Pitch CAS (PID), climb at constant pitch angle -%
    % if ~exist('eI_theta', 'var')
    %     eI_theta = 0;
    % end
    % ut = 1; % full throttle
    % Kp_theta = 1;
    % Ki_theta = 1;
    % Kd_theta = 1;
    % e_theta = deg2rad(20) - theta;
    % eI_theta = eI_theta + Ki_theta*e_theta;
    % eI_theta = min(max(eI_theta,-1),1);
    % ue = Kp_theta*e_theta - Kd_theta*q + eI_theta;
    % ua = -p + ua_in;
    % ur = -r + ur_in;
    
    %- Altitude, climb and level out -%
    % if ~exist('eI_theta', 'var')
    %     eI_theta = 0;
    % end
    % h = -z;
    % h_ref = 3000;
    % h_err = min(max(0.01*(h_ref - h) - 0.01*(-w), -deg2rad(15)), deg2rad(15)); % assumed pitch angle limit at 15 deg
    % Kp_theta = 3;
    % Ki_theta = 0.01;
    % Kd_theta = 2;
    % e_theta = h_err - theta;
    % eI_theta = eI_theta + Ki_theta*e_theta;
    % eI_theta = min(max(eI_theta,-1),1);
    % ue = Kp_theta*e_theta - Kd_theta*q + eI_theta;
    % ut = min(max(3*(h_ref - h), 0), 1);
    % ua = -p + ua_in;
    % ur = -r + ur_in;
    
    %- Roll-Yaw SAS -%
    %- Turn-Coordinator / Emergency Descend -%
    % Kpp = 1; % roll gain
    % Kpd = 1; % rate roll gain
    % phi_ref = deg2rad(30);
    % p_ref   = 0; % reference roll rate command
    % ua = Kpp*(phi_ref - phi) + Kpd*(p_ref - p) + ua_in;
    % 
    % rr = deg2rad(1); % reference yaw rate command
    % Kr = 1; % rate yaw gain
    % ur = Kr*(rr - r) + ur_in;
    % 
    % ue = -q + ue_in;
    % ut = ut_in;
    
    %- Bank-Heading CAS (LQR Full-State Feddback) -%
    %- Forward-slip landing -%
    % phi_ref = deg2rad(30);
    % psi_ref = deg2rad(10);
    % K = [-0.0169   -0.5896   -0.0929   -1.0566   -0.2280
    %       0.3838    0.0128   -1.1973   -0.2366   -0.9737];
    % ua_ur = -K*[0-beta; 0-p; 0-r; phi_ref - phi; psi_ref - psi];
    % ua = ua_ur(1);
    % ur = ua_ur(2);
    % ue = -q + ue_in;
    % ut = ut_in;
    
    %- Velocity Hold -%
    %- Speed Control / Gliding -%
    % if ~exist('eI_theta', 'var')
    %     eI_theta = 0;
    % end
    % if ~exist('eI_u', 'var')
    %     eI_u = 0;
    % end
    % u_ref = 55; % m/s
    % e_u = u_ref - u;
    % eI_u = eI_u + e_u;
    % eI_u = min(max(eI_u,-500),500);
    % ut = min(max(2*e_u + eI_u, 0), 1);
    % 
    % Kp_theta = 1;
    % Ki_theta = 0.01;
    % Kd_theta = 1;
    % e_theta = deg2rad(0) - theta; % level
    % eI_theta = eI_theta + Ki_theta*e_theta;
    % eI_theta = min(max(eI_theta,-1),1);
    % ue = Kp_theta*e_theta - Kd_theta*q + eI_theta;
    % ua = -p + ua_in;
    % ur = -r + ur_in;
    
    %- Altitude Hold Velocity Hold (Cruise Control) -%
    % if ~exist('eI_theta', 'var')
    %     eI_theta = 0;
    % end
    % if ~exist('eI_u', 'var')
    %     eI_u = 0;
    % end
    % h = -z;
    % u_ref = 55; % m/s
    % e_u = u_ref - u;
    % eI_u = eI_u + e_u;
    % eI_u = min(max(eI_u,-500),500);
    % ut = min(max(2*e_u + eI_u, 0), 1);
    % 
    % h_ref = 3000;
    % h_err = min(max(0.01*(h_ref - h) - 0.01*(-w), -deg2rad(15)), deg2rad(15)); % assumed pitch angle limit at 15 deg
    % Kp_theta = 3;
    % Ki_theta = 0.01;
    % Kd_theta = 2;
    % e_theta = h_err - theta;
    % eI_theta = eI_theta + Ki_theta*e_theta;
    % eI_theta = min(max(eI_theta,-1),1);
    % ue = Kp_theta*e_theta - Kd_theta*q + eI_theta;
    % 
    % ua = -p + ua_in;
    % ur = -r + ur_in;

    %% Correct for Actuator Direction
    AileronOut  = -ua;
    ElevatorOut = -ue;
    RudderOut   = -ur;
    ThrottleOut =  ut;
end
